simulink model "v_f_control_system"  (R2019b)
settings: Solver=ode23  StartTime=0.0  StopTime=4  RelTol=1e-3  EnableMultiTasking=on
libraries: powerlib x4, powerlib_extras x1, simulink x1
settings Model: Creator=Administrator  LastModifiedBy=96547
settings DataIOCC: LimitDataPoints=on  SaveFormat=Array  SignalLoggingSaveFormat=ModelDataLogs  ReturnWorkspaceOutputs=off
settings OptimizationCC: ExpressionDepthLimit=2147483647  LifeSpan=inf
settings DebuggingCC: UnderspecifiedInitializationDetection=Classic  MergeDetectMultiDrivingBlocksExec=none  SolverPrmCheckMsg=warning  FcnCallInpInsideContextMsg=warning  StateNameClashWarn=warning  SFUnexpectedBacktrackingDiag=warning  SFNoUnconditionalDefaultTransitionDiag=warning  ArithmeticOperatorsInVariantConditions=warning
settings HardwareCC: ProdBitPerPointer=32  ProdBitPerSizeT=32  ProdBitPerPtrDiffT=32  ProdLargestAtomicFloat=None  ProdIntDivRoundTo=Undefined  ProdEndianess=Unspecified  ProdWordSize=32  ProdHWDeviceType=32-bit Generic
settings ModelReferenceCC: PropagateSignalLabelsOutOfModel=off
settings SFSimCC: SimUseLocalCustomCode=off  CustomCodeUndefinedFunction=UseInterfaceOnly
settings RTWCC: RTWUseLocalCustomCode=off
settings CodeAppCC: StateflowObjectComments=on
settings GRTTargetCC: TargetLangStandard=C89/C90 (ANSI)  GeneratePreprocessorConditionals=Disable all
settings ConfigComp: CovMetricSettings=dw  CovHtmlReporting=on  CovSaveCumulativeToWorkspaceVar=on  CovSaveSingleToWorkspaceVar=on  CovExternalEMLEnable=off
settings SimscapeCC: SimscapeNormalizeSystem=off

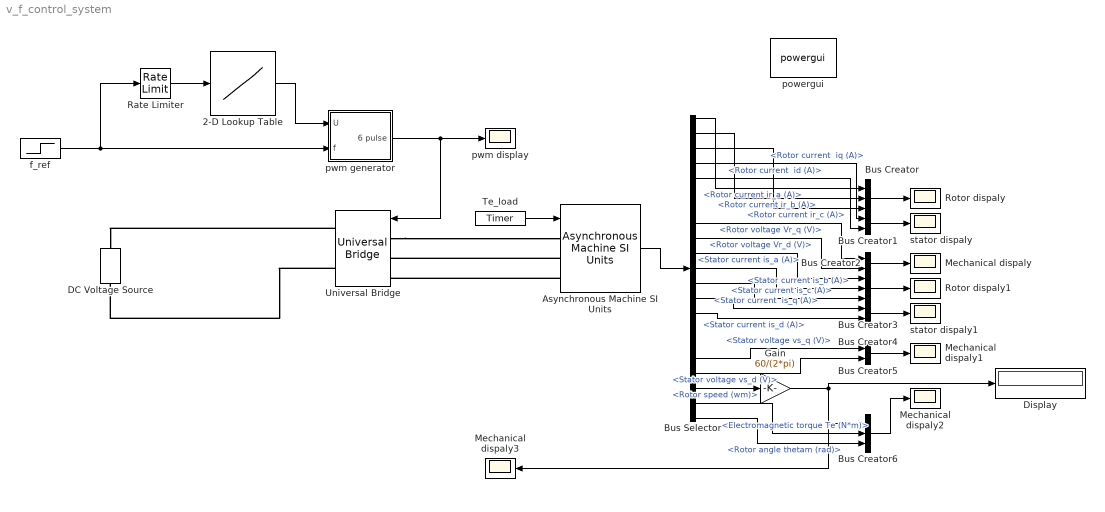
== system v_f_control_system ==
  2-D Lookup Table : Lookup_n-D  NumberOfTableDimensions=1  BreakpointsForDimension1=[0 5 25 50 100]  BreakpointsForDimension2=[1:3]  Table=[0.1 0.1 0.5 1 1]  RndMeth=Simplest  InputSameDT=on
  Asynchronous Machine SI Units : powerlib/Machines/Asynchronous Machine SI Units  RotorType=Squirrel-cage  PresetModel=No  MechanicalLoad=Torque Tm  ShowDetailedParameters=on  ReferenceFrame=Rotor  Units=SI  MeasurementBus=off  NominalParameters=[ 2200, 380, 50 ]  Stator=[ 3.478 0.01254]  Rotor=[ 2.546 0.01226]  Cage1=[ 0.022 0.226/377]  Cage2=[ 0.022 0.226/377]  Lm=0.3329  Mechanical="[ 0.0131  0  2 ]"  PolePairs=2  InitialConditions=[1 0 0 0 0 0 0 0]  SimulateSaturation=off  Saturation=[14.03593122, 27.81365428, 53.79336849, 72.68890987, 97.98006896, 148.6815601, 215.7428561, 302.9841135, 420.4778367 ; 230, 322, 414, 460, 506, 552, 598, 644, 690]  LoadFlowParameters=1492000  TsPowergui=0  TsBlock=-1  IterativeModel=Forward Euler  IterativeDiscreteModel=Trapezoidal non iterative  Pmec=0
      settings: SourceProductName=Simscape Electrical
  Bus Creator : BusCreator  Inputs=3
  Bus Creator{1..2,4..5} (4 alike) : BusCreator  Inputs=2
  Bus Creator3 : BusCreator  Inputs=3
  Bus Creator6 : BusCreator  Inputs=3
  Bus Selector : BusSelector  OutputSignals="Rotor measurements.Rotor current ir_a (A),Rotor measurements.Rotor current ir_b (A),Rotor measurements.Rotor current ir_c (A),Rotor measurements.Rotor current  iq (A),Rotor measurements.Rotor current  id (A),Rotor measurements.Rotor flux phir_q (V s),Rotor measurements.Rotor flux phir_d (V s),Rotor measurements.Rotor voltage Vr_q (V),Rotor measurements.Rotor voltage Vr_d (V),Stator measurements.Stator current is_a (A),Stator measurements.Stator current is_b (A),Stator measurements.Stator current is_c (A),Stator measurements.Stator current  is_q (A),Stator measurements.Stator current is_d (A),Stator measurements.Stator flux phis_q (V s),Stator measurements.Stator flux phis_d (V s),Stator measurements.Stator voltage vs_q (V),Stator measurements.Stator voltage vs_d (V),Mechanical.Rotor speed (wm),Mechanical.Electromagnetic torque Te (N*m),Mechanical.Rotor angle thetam (rad)"
  DC Voltage Source : powerlib/Electrical Sources/DC Voltage Source  Amplitude=621  Measurements=None
      settings: SourceProductName=Simscape Electrical
  Display : Display
  Gain : Gain  Gain=60/(2*pi)
  Mechanical dispaly{,1..3} (4 alike) : Scope
  Rate Limiter : RateLimiter  RisingSlewLimit=200  FallingSlewLimit=-200
  Rotor dispaly : Scope
  Rotor dispaly1 : Scope
  Te_load : powerlib_extras/Control  Blocks/Timer  t="[ 0  0.5  4  ]"  e="[0  14.764 14.764]"
      settings: SourceProductName=Simscape Electrical  SourceProductBaseCode=PS
  Universal Bridge : powerlib/Power Electronics/Universal Bridge  Arms=3  SnubberResistance=1e5  SnubberCapacitance=inf  Device=IGBT / Diodes  Ron=1e-3  Lon=0  ForwardVoltages="[  0  0  ]"  ForwardVoltage=0  GTOparameters=[ 10e-6 , 20e-6 ]  IGBTparameters=[ 1e-6 , 2e-6 ]  Measurements=None  Measurements_2=None  converterType=Rectifier
      settings: SourceProductName=Simscape Electrical
  f_ref : Step  Before=50  After=30  SampleTime=0
  powergui : powerlib/powergui  Priority=1  SimulationMode=Discrete  SampleTime=1e-5  frequency=60  Iterations=50  frequencyindice=50  Pbase=100e6  ErrMax=1e-4  UnitsV=kV  UnitsW=MW  buscounter=0  FunctionMessages=off  echomessages=off  EnableUseOfTLC=off  CurrentSourceSwitches=off  DisableSnubberDevices=off  DisableRonSwitches=off  DisableVfSwitches=off  DisplayEquations=off  AutomaticDiscreteSolvers=off  SolverType=Tustin  Interpol=off  ExternalGateDelay=off  methode=off  Ts=100  x0status=blocks  SPID=off  SwTol=0  HookPort=off  NonlinearTolerance=1e-4  nMaxIteration=100  ContinueOnMaxIteration=off  RestoreLinks=warning  ResistiveCurrentMeasurement=off  Frange=[0:2:500]  Ylog=off  Xlog=on  ShowGrid=off  save=off  variable=ZData  structure=0  ZoomFFT=off  StartTime=0.0  cycles=1  DisplayStyle=1  fundamental=60  FreqAxis=off  MaxFrequency=1000  frequencyindicesteady=1  RmsSteady=1  display=off
      settings: SourceProductName=Simscape Electrical
  pwm display : Scope
  pwm generator : Subsystem
  stator dispaly : Scope
  stator dispaly1 : Scope
  wires:
  pwm generator/1(6 pulse) -> Universal Bridge/1, pwm display/1
  f_ref/1 -> pwm generator/2(f), Rate Limiter/1
  Rate Limiter/1 -> 2-D Lookup Table/1
  2-D Lookup Table/1 -> pwm generator/1(U)
  Te_load/1 -> Asynchronous Machine SI Units/1
  Asynchronous Machine SI Units/1 -> Bus Selector/1
  Bus Selector/1 -> Bus Creator/1  "<Rotor current ir_a (A)>"
  Bus Selector/2 -> Bus Creator/2  "<Rotor current ir_b (A)>"
  Bus Selector/3 -> Bus Creator/3  "<Rotor current ir_c (A)>"
  Bus Creator/1 -> Rotor dispaly/1
  Bus Selector/4 -> Bus Creator1/1  "<Rotor current  iq (A)>"
  Bus Selector/5 -> Bus Creator1/2  "<Rotor current  id (A)>"
  Bus Selector/8 -> Bus Creator2/1  "<Rotor voltage Vr_q (V)>"
  Bus Selector/9 -> Bus Creator2/2  "<Rotor voltage Vr_d (V)>"
  Bus Creator1/1 -> stator dispaly/1
  Bus Creator2/1 -> Mechanical dispaly/1
  Bus Creator3/1 -> Rotor dispaly1/1
  Bus Creator4/1 -> stator dispaly1/1
  Bus Creator5/1 -> Mechanical dispaly1/1
  Bus Selector/10 -> Bus Creator3/1  "<Stator current is_a (A)>"
  Bus Selector/11 -> Bus Creator3/2  "<Stator current is_b (A)>"
  Bus Selector/12 -> Bus Creator3/3  "<Stator current is_c (A)>"
  Bus Selector/13 -> Bus Creator4/1  "<Stator current  is_q (A)>"
  Bus Selector/14 -> Bus Creator4/2  "<Stator current is_d (A)>"
  Bus Selector/17 -> Bus Creator5/1  "<Stator voltage vs_q (V)>"
  Bus Selector/18 -> Bus Creator5/2  "<Stator voltage vs_d (V)>"
  Bus Selector/20 -> Bus Creator6/2  "<Electromagnetic torque Te (N*m)>"
  Bus Selector/21 -> Bus Creator6/3  "<Rotor angle thetam (rad)>"
  Bus Creator6/1 -> Mechanical dispaly2/1
  Bus Selector/19 -> Gain/1  "<Rotor speed (wm)>"
  Gain/1 -> Mechanical dispaly3/1, Bus Creator6/1, Display/1
  connections:
  Universal Bridge/LConn1 -- Asynchronous Machine SI Units/LConn1
  Asynchronous Machine SI Units/LConn2 -- Universal Bridge/LConn2
  Asynchronous Machine SI Units/LConn3 -- Universal Bridge/LConn3
  Universal Bridge/RConn2 -- DC Voltage Source/LConn1
  Universal Bridge/RConn1 -- DC Voltage Source/RConn1

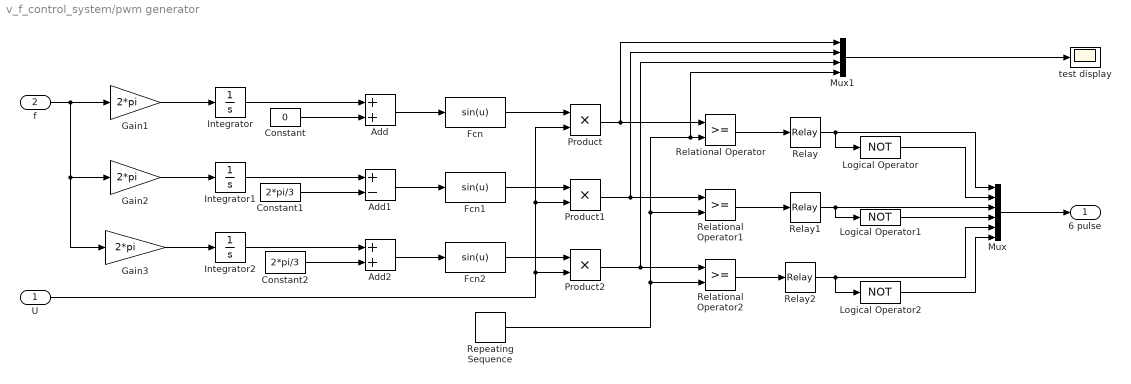
== system v_f_control_system/pwm generator ==
  U : Inport
  f : Inport  Port=2
  Add : Sum
  Add1 : Sum  Inputs=+-
  Add2 : Sum
  Constant : Constant  Value=0
  Constant1 : Constant  Value=2*pi/3
  Constant2 : Constant  Value=2*pi/3
  Fcn : Fcn  Expr=sin(u)
  Fcn1 : Fcn  Expr=sin(u)
  Fcn2 : Fcn  Expr=sin(u)
  Gain1 : Gain  Gain=2*pi
  Gain2 : Gain  Gain=2*pi
  Gain3 : Gain  Gain=2*pi
  Integrator : Integrator
  Integrator1 : Integrator
  Integrator2 : Integrator
  Logical Operator : Logic  Operator=NOT  AllPortsSameDT=off  OutDataTypeStr=boolean
  Logical Operator1 : Logic  Operator=NOT  AllPortsSameDT=off  OutDataTypeStr=boolean
  Logical Operator2 : Logic  Operator=NOT  AllPortsSameDT=off  OutDataTypeStr=boolean
  Mux : Mux  Inputs=6
  Mux1 : Mux
  Product : Product  RndMeth=Zero
  Product1 : Product  RndMeth=Zero
  Product2 : Product  RndMeth=Zero
  Relational Operator : RelationalOperator  OutDataTypeStr=boolean  RndMeth=Nearest
  Relational Operator1 : RelationalOperator  OutDataTypeStr=boolean  RndMeth=Nearest
  Relational Operator2 : RelationalOperator  OutDataTypeStr=boolean  RndMeth=Nearest
  Relay : Relay
  Relay1 : Relay
  Relay2 : Relay
  Repeating Sequence : simulink/Sources/Repeating Sequence  rep_seq_t=[0 0.5/3000 1/3000]  rep_seq_y=[-1 1 -1]
  test display : Scope
  6 pulse : Outport
  wires:
  f/1 -> Gain1/1, Gain3/1, Gain2/1
  Gain1/1 -> Integrator/1
  Gain2/1 -> Integrator1/1
  Gain3/1 -> Integrator2/1
  Integrator/1 -> Add/1
  Integrator1/1 -> Add1/1
  Integrator2/1 -> Add2/1
  Constant/1 -> Add/2
  Constant1/1 -> Add1/2
  Constant2/1 -> Add2/2
  Add/1 -> Fcn/1
  Add1/1 -> Fcn1/1
  Add2/1 -> Fcn2/1
  Repeating Sequence/1 -> Relational Operator2/2, Relational Operator1/2, Relational Operator/2, Mux1/4
  Relational Operator/1 -> Relay/1
  Relational Operator1/1 -> Relay1/1
  Relational Operator2/1 -> Relay2/1
  Mux/1 -> 6 pulse/1
  Fcn/1 -> Product/1
  Fcn2/1 -> Product2/1
  Fcn1/1 -> Product1/1
  U/1 -> Product1/2, Product/2, Product2/2
  Product/1 -> Relational Operator/1, Mux1/1
  Product2/1 -> Relational Operator2/1, Mux1/3
  Product1/1 -> Relational Operator1/1, Mux1/2
  Relay/1 -> Mux/1, Logical Operator/1
  Logical Operator/1 -> Mux/2
  Relay1/1 -> Mux/3, Logical Operator1/1
  Logical Operator1/1 -> Mux/4
  Relay2/1 -> Mux/5, Logical Operator2/1
  Logical Operator2/1 -> Mux/6
  Mux1/1 -> test display/1
